simulink model "step_response_open_loop"  (R2023a)
settings: Solver=VariableStepAuto  StartTime=0.0  StopTime=t_simulation  RelTol=1e-3
undefined symbols (not defined in the file or in its folder): simP
settings Model: Creator=pascalbock  LastModifiedBy=pascalbock

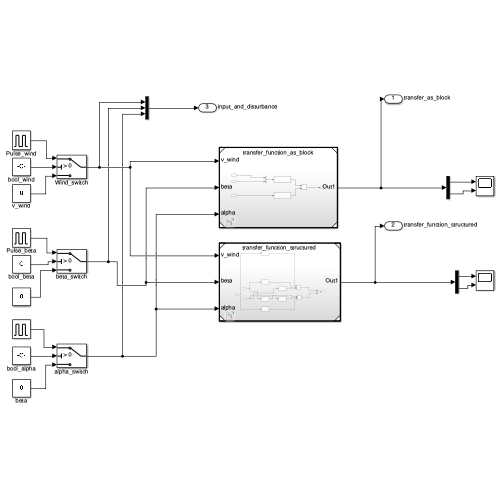
[thumbnail: Simulink's stored preview of the top-level diagram]
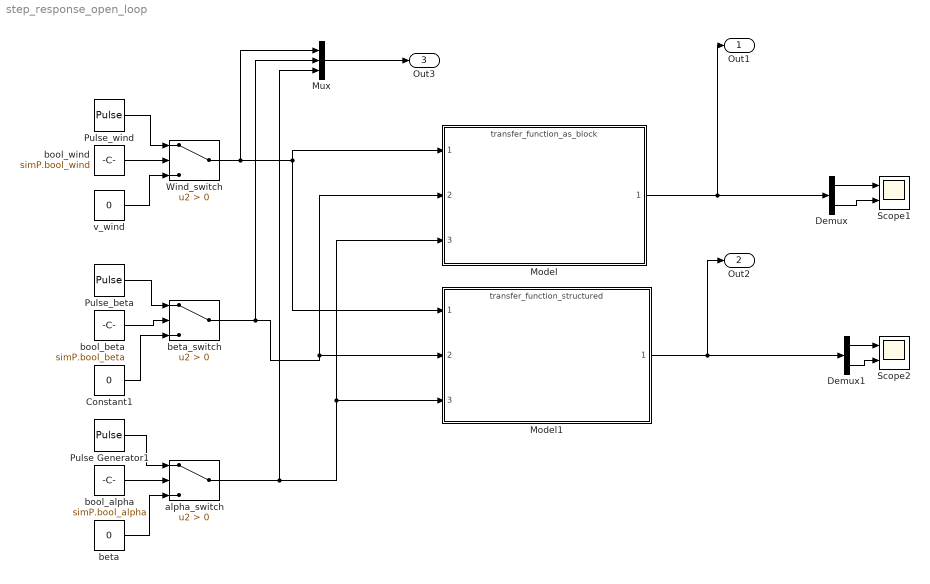
== system step_response_open_loop ==
  Constant1 : Constant  Value=0
  Demux : Demux  Outputs=2
  Demux1 : Demux  Outputs=2
  Model : ModelReference  ModelNameDialog=transfer_function_as_block.slx  SimulationMode=Normal  ModelReferenceVersion=1.3
  Model1 : ModelReference  ModelNameDialog=transfer_function_structured.slx  SimulationMode=Normal  ModelReferenceVersion=1.1
  Mux : Mux  Inputs=3
  Pulse Generator1 : DiscretePulseGenerator  PulseType=Time based  Amplitude=simP.A_alpha  Period=simP.T_period  PulseWidth=simP.pulse_width  PhaseDelay=simP.T_delay
  Pulse_beta : DiscretePulseGenerator  PulseType=Time based  Amplitude=simP.A_beta  Period=simP.T_period  PulseWidth=simP.pulse_width  PhaseDelay=simP.T_delay
  Pulse_wind : DiscretePulseGenerator  PulseType=Time based  Amplitude=simP.A_wind  Period=simP.T_period  PulseWidth=simP.pulse_width  PhaseDelay=simP.T_delay
  Scope1 : Scope  NumInputPorts=2
  Scope2 : Scope  NumInputPorts=2
  Wind_switch : Switch  Criteria=u2 > Threshold  SaturateOnIntegerOverflow=off  InputSameDT=off
  alpha_switch : Switch  Criteria=u2 > Threshold  SaturateOnIntegerOverflow=off  InputSameDT=off
  beta : Constant  Value=0
  beta_switch : Switch  Criteria=u2 > Threshold  SaturateOnIntegerOverflow=off  InputSameDT=off
  bool_alpha : Constant  Value=simP.bool_alpha
  bool_beta : Constant  Value=simP.bool_beta
  bool_wind : Constant  Value=simP.bool_wind
  v_wind : Constant  Value=0
  Out1 : Outport  SignalName=transfer_as_block
  Out2 : Outport  Port=2  SignalName=transfer_function_structured
  Out3 : Outport  Port=3  SignalName=input_and_disturbance
  wires:
  Model/1 -> Out1/1, Demux/1
  Demux/1 -> Scope1/1
  Demux/2 -> Scope1/2
  Pulse_wind/1 -> Wind_switch/1
  v_wind/1 -> Wind_switch/3
  bool_wind/1 -> Wind_switch/2
  bool_alpha/1 -> alpha_switch/2
  beta/1 -> alpha_switch/3
  Pulse_beta/1 -> beta_switch/1
  Pulse Generator1/1 -> alpha_switch/1
  bool_beta/1 -> beta_switch/2
  Wind_switch/1 -> Mux/1, Model1/1, Model/1
  alpha_switch/1 -> Mux/3, Model1/3, Model/3
  Constant1/1 -> beta_switch/3
  Model1/1 -> Out2/1, Demux1/1
  Demux1/1 -> Scope2/1
  Demux1/2 -> Scope2/2
  beta_switch/1 -> Mux/2, Model1/2, Model/2
  Mux/1 -> Out3/1
